simulink model "AnesthesiaMachine"  (R2024b)
settings: Solver=VariableStepAuto  StartTime=0.0  StopTime=10.0  RelTol=1e-3
settings Model: Creator=Hp  LastModifiedBy=Hp

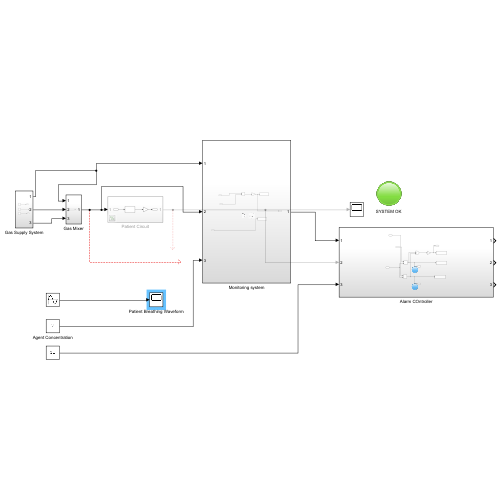
[thumbnail: Simulink's stored preview of the top-level diagram]
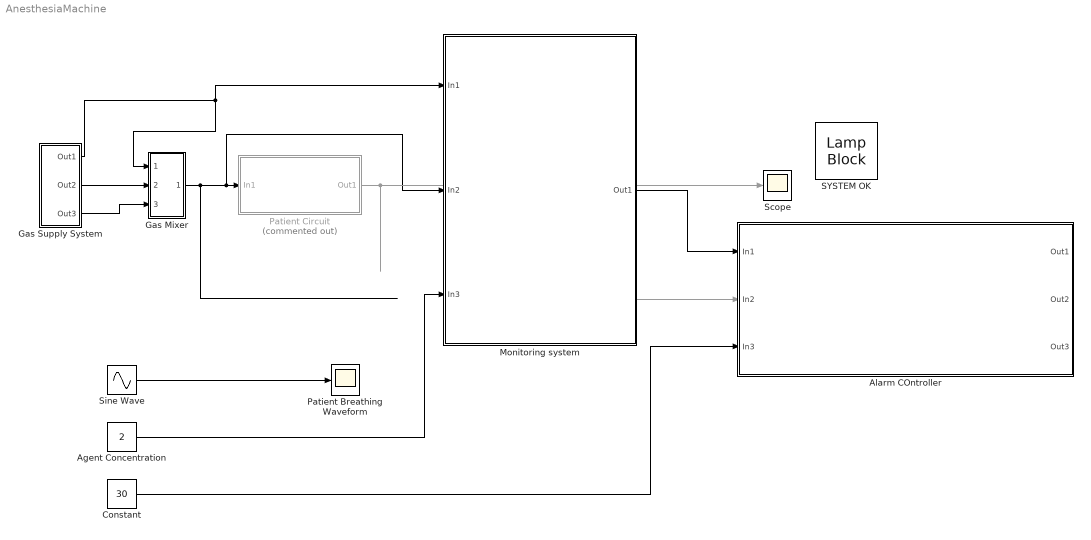
== system AnesthesiaMachine ==
  Agent Concentration : Constant  Value=2
  Alarm COntroller : Subsystem
  Constant : Constant  Value=30
  Gas Mixer : Subsystem
  Gas Supply System : Subsystem
  Monitoring system : Subsystem
  Patient Breathing Waveform : Scope
  Patient Circuit : Subsystem  Commented=on
  SYSTEM OK : LampBlock  LabelPosition=Hide
  Scope : Scope
  Sine Wave : Sin  Frequency=1.5  SampleTime=0
  wires:
  Sine Wave/1 -> Patient Breathing Waveform/1
  Gas Supply System/1(Out1) -> Monitoring system/1(In1), Gas Mixer/1(In1)
  Gas Mixer/1(Out1) -> Monitoring system/2(In2), Patient Circuit/1(In1)
  Gas Supply System/2(Out2) -> Gas Mixer/2(In2)
  Gas Supply System/3(Out3) -> Gas Mixer/3(In3)
  Patient Circuit/1(Out1) -> Alarm COntroller/2(In2), Scope/1
  Constant/1 -> Alarm COntroller/3(In3)
  Agent Concentration/1 -> Monitoring system/3(In3)
  Monitoring system/1(Out1) -> Alarm COntroller/1(In1)

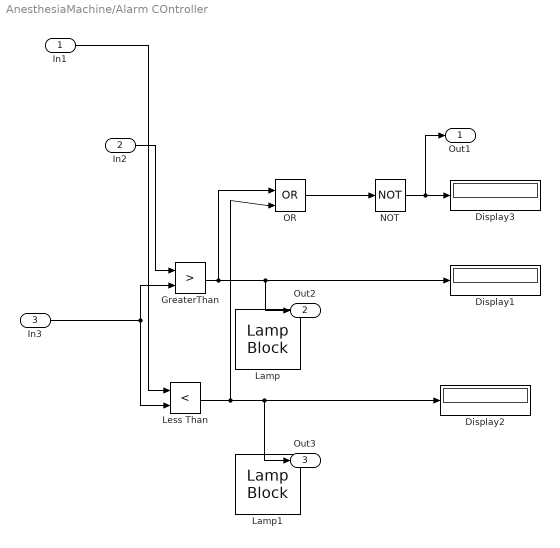
== system AnesthesiaMachine/Alarm COntroller ==
  In1 : Inport
  In2 : Inport  Port=2
  In3 : Inport  Port=3
  Display1 : Display
  Display2 : Display
  Display3 : Display
  GreaterThan : RelationalOperator  Operator=>  OutDataTypeStr=boolean  RndMeth=Simplest
  Lamp : LampBlock  LabelPosition=Hide
  Lamp1 : LampBlock  LabelPosition=Hide
  Less Than : RelationalOperator  Operator=<  OutDataTypeStr=boolean  RndMeth=Simplest  InputSameDT=off
  NOT : Logic  Operator=NOT  IconShape=distinctive  AllPortsSameDT=off  OutDataTypeStr=boolean
  OR : Logic  Operator=OR  IconShape=distinctive  AllPortsSameDT=off  OutDataTypeStr=boolean
  Out1 : Outport
  Out2 : Outport  Port=2
  Out3 : Outport  Port=3
  wires:
  In2/1 -> GreaterThan/1
  OR/1 -> NOT/1
  GreaterThan/1 -> OR/1, Out2/1, Display1/1
  Less Than/1 -> OR/2, Out3/1, Display2/1
  In3/1 -> GreaterThan/2, Less Than/2
  NOT/1 -> Out1/1, Display3/1
  In1/1 -> Less Than/1

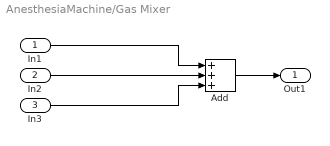
== system AnesthesiaMachine/Gas Mixer ==
  In1 : Inport
  In2 : Inport  Port=2
  In3 : Inport  Port=3
  Add : Sum  Inputs=+++
  Out1 : Outport
  wires:
  In1/1 -> Add/1
  In3/1 -> Add/3
  In2/1 -> Add/2
  Add/1 -> Out1/1

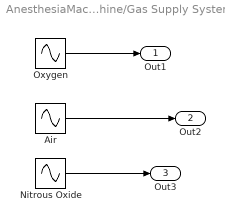
== system AnesthesiaMachine/Gas Supply System ==
  Air : Sin  Amplitude=0.1  Bias=3  Frequency=0.3  SampleTime=0
  Nitrous Oxide : Sin  Amplitude=0.15  Bias=1  Frequency=0.5  SampleTime=0
  Oxygen : Sin  Amplitude=0.2  Bias=2  Frequency=0.2  SampleTime=0
  Out1 : Outport
  Out2 : Outport  Port=2
  Out3 : Outport  Port=3
  wires:
  Oxygen/1 -> Out1/1
  Air/1 -> Out2/1
  Nitrous Oxide/1 -> Out3/1

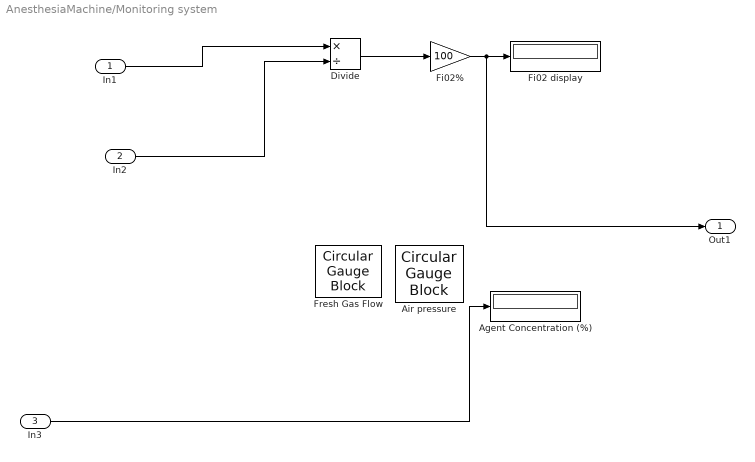
== system AnesthesiaMachine/Monitoring system ==
  In1 : Inport
  In2 : Inport  Port=2
  In3 : Inport  Port=3
  Agent Concentration (%) : Display
  Air pressure : CircularGaugeBlock  ScaleMax=70
  Divide : Product  Inputs=*/
  Fi02 display : Display
  Fi02% : Gain  Gain=100
  Fresh Gas Flow : CircularGaugeBlock  ScaleMax=20
  Out1 : Outport
  wires:
  Divide/1 -> Fi02%/1
  In3/1 -> Agent Concentration (%)/1
  Fi02%/1 -> Out1/1, Fi02 display/1
  In1/1 -> Divide/1
  In2/1 -> Divide/2

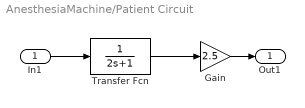
== system AnesthesiaMachine/Patient Circuit ==
  In1 : Inport
  Gain : Gain  Gain=2.5
  Transfer Fcn : TransferFcn  Denominator=[2 1]
  Out1 : Outport
  wires:
  Transfer Fcn/1 -> Gain/1
  Gain/1 -> Out1/1
  In1/1 -> Transfer Fcn/1
